simulink model "SimModel2"  (R2015b)
settings: Solver=ode23s  StartTime=0.0  StopTime=10.0  RelTol=1e-3
values from neighbouring files (symbols this model uses):
  A = [ 0 1; 0 -d/m]    [Exercise1.m]
  B = [0 ; 1/m]    [Exercise1.m]
  C1 = [ 1 0]    [Exercise1.m]
  C2 = [0 1]    [Exercise1.m]
  d = 0.5    [Exercise1.m]
  D = 0    [Exercise1.m]
  Freq = 10    [Exercise1.m]
  m = 0.1    [Exercise1.m]
  Sine_wave = 1    [Exercise1.m]
undefined symbols (not defined in the file or in its folder): G1den, G1num, G2den, G2num, k
libraries: simulink x1
settings Model: Creator=ooman  LastModifiedBy=sofianh

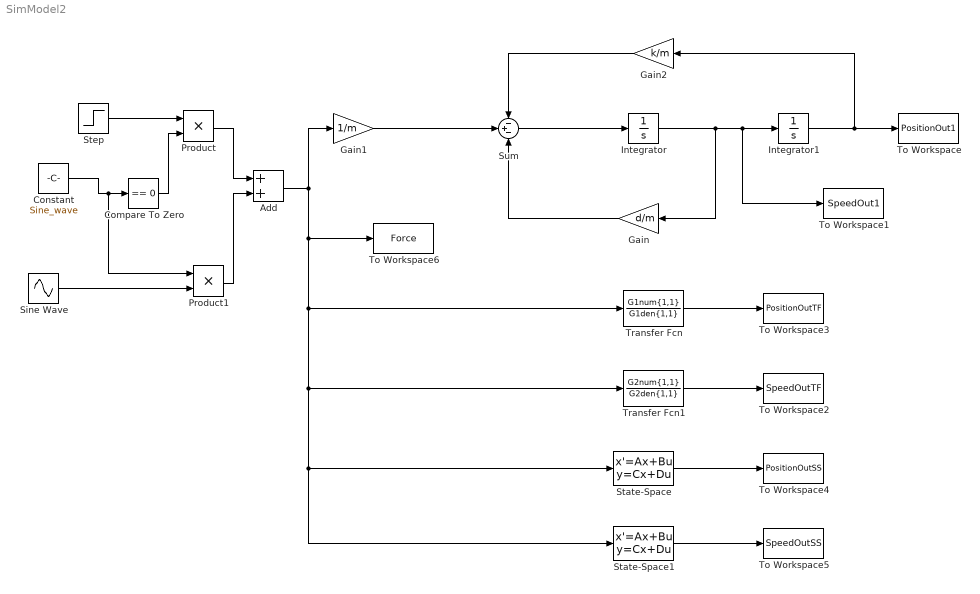
== system SimModel2 ==
  Add : Sum
  Compare To Zero : simulink/Logic and Bit Operations/Compare To Zero  relop===  OutDataTypeStr=boolean
  Constant : Constant  Value=Sine_wave
  Gain : Gain  Gain=d/m
  Gain1 : Gain  Gain=1/m
  Gain2 : Gain  Gain=k/m
  Integrator : Integrator
  Integrator1 : Integrator
  Product : Product
  Product1 : Product
  Sine Wave : Sin  Frequency=Freq  SampleTime=0
  State-Space : StateSpace  A=A  B=B  C=C1  D=D  X0=0  ContinuousStateAttributes='Position'
  State-Space1 : StateSpace  A=A  B=B  C=C2  D=D  X0=0  ContinuousStateAttributes='Speed'
  Step : Step  Time=0  SampleTime=0
  Sum : Sum  Inputs=-+-
  To Workspace : ToWorkspace  VariableName=PositionOut1  SaveFormat=Structure With Time  SampleTime=-1
  To Workspace1 : ToWorkspace  VariableName=SpeedOut1  SaveFormat=Structure With Time  SampleTime=-1
  To Workspace2 : ToWorkspace  VariableName=SpeedOutTF  SaveFormat=Structure With Time  SampleTime=-1
  To Workspace3 : ToWorkspace  VariableName=PositionOutTF  SaveFormat=Structure With Time  SampleTime=-1
  To Workspace4 : ToWorkspace  VariableName=PositionOutSS  SaveFormat=Structure With Time  SampleTime=-1
  To Workspace5 : ToWorkspace  VariableName=SpeedOutSS  SaveFormat=Structure With Time  SampleTime=-1
  To Workspace6 : ToWorkspace  VariableName=Force  SaveFormat=Structure With Time  SampleTime=-1
  Transfer Fcn : TransferFcn  Numerator=G1num{1,1}  Denominator=G1den{1,1}  ContinuousStateAttributes='Position'
  Transfer Fcn1 : TransferFcn  Numerator=G2num{1,1}  Denominator=G2den{1,1}  ContinuousStateAttributes='Speed'
  wires:
  Integrator/1 -> Gain/1, To Workspace1/1, Integrator1/1
  Sum/1 -> Integrator/1
  Integrator1/1 -> Gain2/1, To Workspace/1
  Transfer Fcn/1 -> To Workspace3/1
  Transfer Fcn1/1 -> To Workspace2/1
  State-Space/1 -> To Workspace4/1
  State-Space1/1 -> To Workspace5/1
  Step/1 -> Product/1
  Constant/1 -> Product1/1, Compare To Zero/1
  Sine Wave/1 -> Product1/2
  Product/1 -> Add/1
  Product1/1 -> Add/2
  Add/1 -> Gain1/1, To Workspace6/1, State-Space1/1, State-Space/1, Transfer Fcn1/1, Transfer Fcn/1
  Compare To Zero/1 -> Product/2
  Gain1/1 -> Sum/2
  Gain2/1 -> Sum/1
  Gain/1 -> Sum/3
